simulink model "statefdbk"  (R2021a)
settings: Solver=VariableStepAuto  StartTime=0.0  StopTime=10.0  RelTol=1e-3
values from neighbouring files (symbols this model uses):
  K = lqr(A, B, Qr, Rr)    [Exe1-old.m]    (also in Exe1.m)
  x0 = [0.1 0 0 0 0]'    [Exe1-old.m]    (also in Exe1.m)
undefined symbols (not defined in the file or in its folder): A, B, C, D
settings Model: Creator=Tiago  LastModifiedBy=Tiago

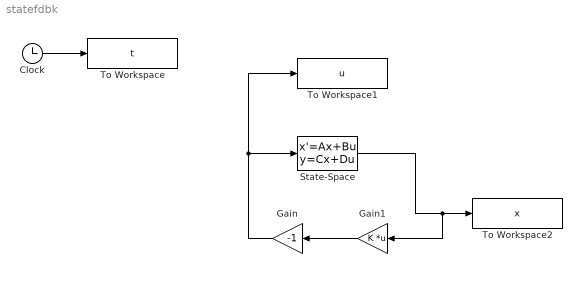
== system statefdbk ==
  Clock : Clock
  Gain : Gain  Gain=-1
  Gain1 : Gain  Gain=K  Multiplication=Matrix(K*u) (u vector)
  State-Space : StateSpace  A=A  B=B  C=C  D=D  InitialCondition=x0
  To Workspace : ToWorkspace  VariableName=t  SaveFormat=Timeseries  SampleTime=-1
  To Workspace1 : ToWorkspace  VariableName=u  SaveFormat=Timeseries  SampleTime=-1
  To Workspace2 : ToWorkspace  VariableName=x  SaveFormat=Timeseries  SampleTime=-1
  wires:
  Clock/1 -> To Workspace/1
  Gain1/1 -> Gain/1
  State-Space/1 -> Gain1/1, To Workspace2/1
  Gain/1 -> To Workspace1/1, State-Space/1
